simulink model "Simulink_Com_Restricao"  (Simulink 8.2)
settings: Solver=ode4  SolverMode=SingleTasking  StartTime=0.0  StopTime=20  FixedStep=0.01  RelTol=1e-3
InitFcn:
  | Main_Simulink_Com_Restricao;
undefined symbols (not defined in the file or in its folder): A1, B1, C, D, T, xk0
undefined symbols (not defined in the file): A, B, Umax
settings Model: Creator=Kawakami  LastModifiedBy=Eduardo  CovHTMLOptions=-sRT=1 -aTS=1 -bRG=1 -bTC=1 -hTR=0 -nFC=0 -scm=1 -bcm=1 -xEv=0  CovNameIncrementing=on
settings DataIOCC: LimitDataPoints=off  SaveOutput=off  SaveTime=off  TimeSaveName=t  SignalLoggingName=sigsOut
settings OptimizationCC: BooleanDataType=off
settings DebuggingCC: SaveWithParameterizedLinksMsg=none  SignalResolutionControl=TryResolveAllWithWarning  SolverPrmCheckMsg=none  MultiTaskDSMMsg=warning  MultiTaskCondExecSysMsg=none
settings HardwareCC: TargetUnknown=on
settings RTWCC: IncludeERTFirstTime=on

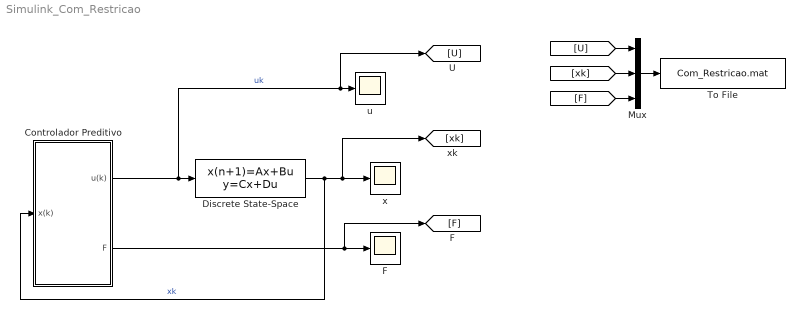
== system Simulink_Com_Restricao ==
  "Controlador Preditivo  " : Subsystem  mask{A=A, B=B, Umax=Umax, T=T}
      mask prompts: A "Matriz Agregada A"; B "Matriz Agregada B"; Umax "Input Max"; T "T (passo da simulação)"
  Discrete State-Space : DiscreteStateSpace  A=A1  B=B1  C=C  D=D  X0=xk0
  F : Scope
      settings: YMin=-1.25  YMax=2.25  SaveName=ScopeData2
  Mux : Mux  Inputs=3
  To File : ToFile  Filename=Com_Restricao.mat  MatrixName=ComRestricao
  u : Scope
      settings: TimeRange=10  YMin=-2  YMax=0.5
  x : Scope
      settings: YMin=-1.25  YMax=2.25
  wires:
  "Controlador Preditivo  "/1(u(k)) -> Discrete State-Space/1, [U], u/1  "uk"
  Discrete State-Space/1 -> "Controlador Preditivo  "/1(x(k)), x/1, [xk]  "xk"
  "Controlador Preditivo  "/2(F) -> [F], F/1
  Mux/1 -> To File/1
  [F] -> Mux/3
  [xk] -> Mux/2
  [U] -> Mux/1

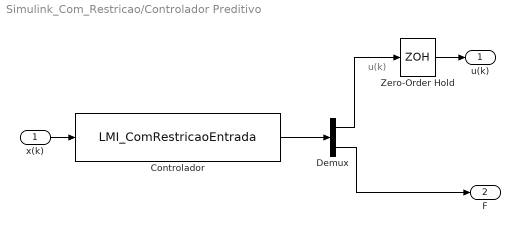
== system Simulink_Com_Restricao/Controlador Preditivo   ==
  note: u(k)
  x(k) : Inport
  Controlador : S-Function  FunctionName=LMI_ComRestricaoEntrada  Parameters=A, B, Umax, T  EnableBusSupport=off
  Demux : Demux  Outputs=2
  Zero-Order Hold : ZeroOrderHold  SampleTime=T
  u(k) : Outport
  F : Outport  Port=2
  wires:
  Zero-Order Hold/1 -> u(k)/1
  x(k)/1 -> Controlador/1
  Controlador/1 -> Demux/1
  Demux/1 -> Zero-Order Hold/1
  Demux/2 -> F/1
